simulink model "TBS_SIM"  (R2021a)
settings: Solver=ode5  StartTime=15  StopTime=100  FixedStep=0.002  RelTol=1e-3
PreLoadFcn:
  | TBS_Cai_simu_init_20170316
StopFcn:
  | TBS_SIMULATION_LOG
undefined symbols (not defined in the file): air_density, g, L1X, L2X, L2Y, L3X, L3Y, MAC1, MAC2, MAC3, magnitude, mass, motor_m0, motor_t0, ORIGIN_CD, ORIGIN_CL, ORIGIN_CM, S_seg1, S_seg2, S_seg3
libraries: aerolibconvert2 x20, pid_lib x10, sharedtransform x4, aerolibwind2 x3, simulink x2, shared6dof x1, aerolibasang x1
(part 3 of 3)

== system TBS_SIM/Variant Control System/Transition/Trans/Cruise Controller/Cruise ==
  Ve : Inport
  Xe : Inport  Port=2
  DCM : Inport  Port=3
  pqr : Inport  Port=4
  V_b : Inport  Port=5
  Euler : Inport  Port=6
  Angle Conversion : aerolibconvert2/Angle Conversion  IU=rad  OU=deg
  Demux : Demux
  Demux2 : Demux  Outputs=3
  Mux1 : Mux  Inputs=2
  Mux3 : Mux  Inputs=2
  Saturation : Saturate  UpperLimit=10000  LowerLimit=0
  Saturation1 : Saturate  UpperLimit=10000  LowerLimit=0
  Saturation2 : Saturate  UpperLimit=16.5  LowerLimit=-23
  Saturation3 : Saturate  UpperLimit=16.5  LowerLimit=-23
  Terminator : Terminator
  map : MATLAB Function  TreatAsAtomicUnit=on
  nav : MATLAB Function  TreatAsAtomicUnit=on
  ve : Scope  NumInputPorts=3
  RS : Outport
  "Actuator " : Outport  Port=2
  wires:
  V_b/1 -> nav/3(v)
  map/1(output) -> Demux/1
  Saturation/1 -> Mux1/1
  Demux/1 -> Saturation/1
  Demux/2 -> Saturation1/1
  Saturation1/1 -> Mux1/2
  Saturation2/1 -> Mux3/1
  Demux/4 -> Saturation3/1
  Saturation3/1 -> Mux3/2
  Demux/3 -> Saturation2/1
  nav/1(output) -> map/1(F_des)
  Angle Conversion/1 -> nav/2(PRY)
  Demux2/1 -> ve/1
  Demux2/2 -> ve/2
  Demux2/3 -> ve/3
  Ve/1 -> Demux2/1
  Xe/1 -> nav/1(p)
  pqr/1 -> nav/4(pqr)
  Mux1/1 -> RS/1
  Mux3/1 -> "Actuator "/1
  Euler/1 -> Angle Conversion/1
  DCM/1 -> Terminator/1

== system TBS_SIM/Variant Control System/Transition/Trans/Transition Controller/Hover ==
  Ve : Inport
  Xe : Inport  Port=2
  DCM : Inport  Port=3
  pqr : Inport  Port=4
  des_v : Inport  Port=5
  des_p : Inport  Port=6
  Attitude controller : Subsystem
  Constant1 : Constant  Value=[0,0,0]
  Demux4 : Demux
  Direction Cosine Matrix to Rotation Angles : sharedtransform/Direction Cosine Matrix to Rotation Angles  rotationOrder=YZX  aMode=aMode  action=None  tolerance=eps(2)
      settings: SourceProductBaseCode=AE,PW,DR,MT,UV,VE
  Mux2 : Mux  Inputs=2
  Mux4 : Mux  Inputs=2
  Nav_controller(quad_axes) : Subsystem
  Ramp1 : simulink/Sources/Ramp  slope=18  start=0  InitialOutput=0
  Saturation1 : Saturate  UpperLimit=80
  Saturation4 : Saturate  UpperLimit=10000  LowerLimit=0
  Saturation5 : Saturate  UpperLimit=10000  LowerLimit=0
  Saturation6 : Saturate  UpperLimit=16.5  LowerLimit=-23
  Saturation7 : Saturate  UpperLimit=16.5  LowerLimit=-23
  Scope : Scope  NumInputPorts=2
  Sum : Sum  Inputs=-+|
  map1 : Subsystem
  RS : Outport
  "Actuator " : Outport  Port=2
  wires:
  Saturation6/1 -> Mux4/1
  map1/1(Act) -> Demux4/1
  Mux4/1 -> "Actuator "/1
  Saturation4/1 -> Mux2/1
  Ve/1 -> Nav_controller(quad_axes)/1(True velocity)
  Demux4/2 -> Saturation5/1
  Demux4/4 -> Saturation7/1
  Saturation7/1 -> Mux4/2
  Xe/1 -> Nav_controller(quad_axes)/2(True Position)
  Demux4/1 -> Saturation4/1
  Saturation5/1 -> Mux2/2
  DCM/1 -> Direction Cosine Matrix to Rotation Angles/1
  Nav_controller(quad_axes)/1(phi_des) -> Attitude controller/1(phi_des)
  Attitude controller/2("M_C ") -> map1/2(M_c)
  Demux4/3 -> Saturation6/1
  pqr/1 -> Attitude controller/5(pqr)
  Direction Cosine Matrix to Rotation Angles/1 -> Nav_controller(quad_axes)/5(True PRY), Attitude controller/4(PRY)
  Attitude controller/1(F_c) -> map1/1(F_c)
  Constant1/1 -> Attitude controller/6(des_pqr)
  Nav_controller(quad_axes)/3(F_des) -> Attitude controller/3(F_des)
  Mux2/1 -> RS/1
  des_v/1 -> Nav_controller(quad_axes)/3(Desired velocity)
  des_p/1 -> Nav_controller(quad_axes)/4(Desired Position)
  Saturation1/1 -> Sum/1
  Ramp1/1 -> Saturation1/1
  Nav_controller(quad_axes)/2("theta_des ") -> Scope/2, Sum/2  "before slope"
  Sum/1 -> Scope/1, Attitude controller/2(theta_des)  "Theta_des"

== system TBS_SIM/Variant Control System/Transition/Trans/Transition Controller/Hover/Attitude controller ==
  phi_des : Inport
  theta_des : Inport  Port=2
  F_des : Inport  Port=3
  PRY : Inport  Port=4
  pqr : Inport  Port=5
  des_pqr : Inport  Port=6
  Add : Sum  Inputs=+-
  Angle Conversion1 : aerolibconvert2/Angle Conversion  IU=rad  OU=deg
  Constant1 : Constant  Value=90
  Demux : Demux  Outputs=3
  Gain : Gain  Gain=[-0.05;0.07;0.08]
  Gain1 : Gain  Gain=[-0.4;-0.8;1.4]
  Gain2 : Gain  Gain=[0 0 1; 0 1 0; 1 0 0]  Multiplication=Matrix(K*u)
  Gain3 : Gain  Gain=-1
  Gain4 : Gain  Gain=-1
  Mux : Mux  Inputs=3
  Scope1 : Scope
  Scope2 : Scope
  error_phi : Sum  Inputs=-+
  error_phi1 : Sum  Inputs=-+
  error_pqr : Sum  Inputs=-+
  error_pqr1 : Sum  Inputs=-+
  F_c : Outport
  "M_C " : Outport  Port=2
  wires:
  F_des/1 -> F_c/1
  des_pqr/1 -> error_pqr/1
  pqr/1 -> error_pqr/2
  phi_des/1 -> error_phi/1
  theta_des/1 -> error_phi1/1
  error_phi1/1 -> Mux/2
  Gain/1 -> Add/1
  Gain1/1 -> Scope2/1, Add/2
  PRY/1 -> Angle Conversion1/1
  error_phi/1 -> Mux/1
  Gain4/1 -> Mux/3
  Mux/1 -> Scope1/1, Gain/1
  error_pqr/1 -> Gain2/1
  Gain2/1 -> Gain1/1
  Add/1 -> "M_C "/1
  Demux/2 -> Gain3/1
  Gain3/1 -> error_phi/2
  Demux/1 -> error_pqr1/2
  Constant1/1 -> error_pqr1/1
  error_pqr1/1 -> error_phi1/2
  Angle Conversion1/1 -> Demux/1
  Demux/3 -> Gain4/1

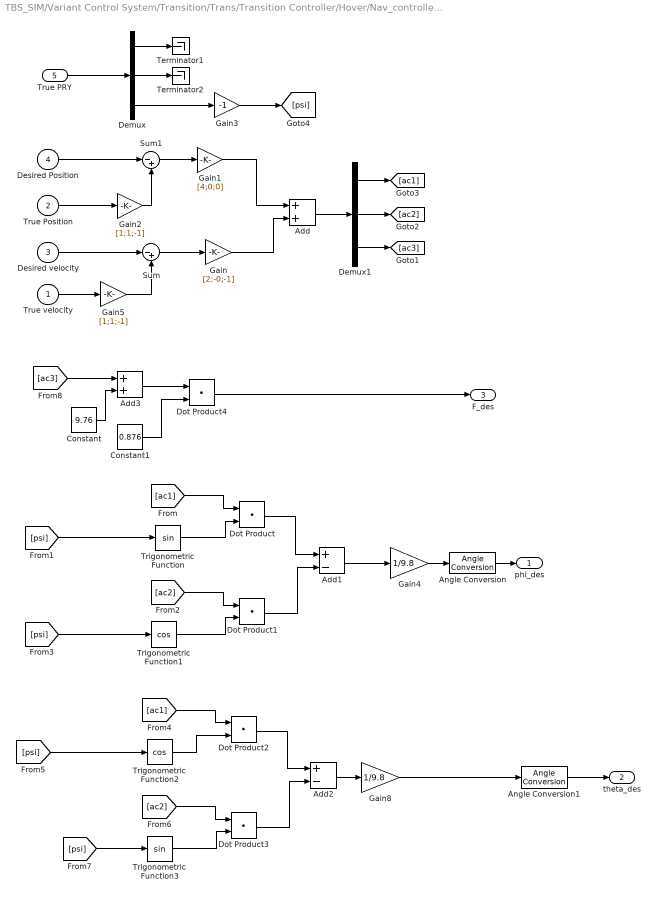
== system TBS_SIM/Variant Control System/Transition/Trans/Transition Controller/Hover/Nav_controller(quad_axes) ==
  True velocity : Inport
  True Position : Inport  Port=2
  Desired velocity : Inport  Port=3
  Desired Position : Inport  Port=4
  True PRY : Inport  Port=5
  Add : Sum
  Add1 : Sum  Inputs=+-
  Add2 : Sum  Inputs=+-
  Add3 : Sum
  Angle Conversion : aerolibconvert2/Angle Conversion  IU=rad  OU=deg
  Angle Conversion1 : aerolibconvert2/Angle Conversion  IU=rad  OU=deg
  Constant : Constant  Value=9.76
  Constant1 : Constant  Value=0.876
  Demux : Demux  Outputs=3
  Demux1 : Demux  Outputs=3
  Dot Product{,1..4} (5 alike) : DotProduct  InputSameDT=on  OutDataTypeStr=Inherit: Inherit via internal rule
  Gain : Gain  Gain=[2;-0;-1]
  Gain1 : Gain  Gain=[4;0;0]
  Gain2 : Gain  Gain=[1;1;-1]
  Gain3 : Gain  Gain=-1
  Gain4 : Gain  Gain=1/9.8
  Gain5 : Gain  Gain=[1;1;-1]
  Gain8 : Gain  Gain=1/9.8
  Sum : Sum  Inputs=|-+
  Sum1 : Sum  Inputs=|-+
  Terminator1 : Terminator
  Terminator2 : Terminator
  Trigonometric Function : Trigonometry
  Trigonometric Function1 : Trigonometry  Operator=cos
  Trigonometric Function2 : Trigonometry  Operator=cos
  Trigonometric Function3 : Trigonometry
  phi_des : Outport
  "theta_des " : Outport  Port=2
  F_des : Outport  Port=3
  wires:
  True velocity/1 -> Gain5/1
  Desired velocity/1 -> Sum/1
  Sum/1 -> Gain/1
  Sum1/1 -> Gain1/1
  Gain1/1 -> Add/1
  Gain/1 -> Add/2
  True PRY/1 -> Demux/1
  Demux/1 -> Terminator1/1
  Demux/3 -> Gain3/1
  Demux/2 -> Terminator2/1
  Add/1 -> Demux1/1
  Demux1/2 -> [ac2]
  [ac1] -> Dot Product/1
  Trigonometric Function/1 -> Dot Product/2
  [psi] -> Trigonometric Function/1
  [ac2] -> Dot Product1/1
  Trigonometric Function1/1 -> Dot Product1/2
  [psi] -> Trigonometric Function1/1
  Dot Product/1 -> Add1/1
  Dot Product1/1 -> Add1/2
  Add1/1 -> Gain4/1
  [ac1] -> Dot Product2/1
  Trigonometric Function2/1 -> Dot Product2/2
  [psi] -> Trigonometric Function2/1
  [ac2] -> Dot Product3/1
  Trigonometric Function3/1 -> Dot Product3/2
  [psi] -> Trigonometric Function3/1
  Dot Product2/1 -> Add2/1
  Dot Product3/1 -> Add2/2
  Add2/1 -> Gain8/1
  [ac3] -> Add3/1
  Constant/1 -> Add3/2
  Add3/1 -> Dot Product4/1
  Constant1/1 -> Dot Product4/2
  Dot Product4/1 -> F_des/1
  Demux1/1 -> [ac1]
  Demux1/3 -> [ac3]
  True Position/1 -> Gain2/1
  Gain2/1 -> Sum1/2
  Desired Position/1 -> Sum1/1
  Gain3/1 -> [psi]
  Gain4/1 -> Angle Conversion/1
  Angle Conversion/1 -> phi_des/1
  Gain8/1 -> Angle Conversion1/1
  Angle Conversion1/1 -> "theta_des "/1
  Gain5/1 -> Sum/2

== system TBS_SIM/Variant Control System/Transition/Trans/Transition Controller/Hover/map1 ==
  F_c : Inport
  M_c : Inport  Port=2
  Constant : Constant  Value=100
  Constant1 : Constant  Value=9.5
  Constant2 : Constant  Value=0.3
  Demux : Demux  Outputs=3
  Gain : Gain  Gain=1000
  Gain1 : Gain  Gain=1000
  Gain2 : Gain  Gain=50
  Gain3 : Gain  Gain=50
  Mux : Mux
  Sum : Sum  Inputs=-+|
  Sum1 : Sum  Inputs=|++
  Sum2 : Sum  Inputs=|+-
  Sum3 : Sum  Inputs=-+|
  Sum4 : Sum  Inputs=|++
  Sum5 : Sum  Inputs=|++
  Sum6 : Sum  Inputs=+-|
  Act : Outport
  wires:
  M_c/1 -> Demux/1
  F_c/1 -> Gain/1
  Demux/1 -> Gain1/1
  Gain1/1 -> Sum/2
  Constant/1 -> Sum/1
  Gain/1 -> Sum2/1, Sum1/1
  Sum/1 -> Sum1/2, Sum2/2
  Sum1/1 -> Mux/1
  Sum2/1 -> Mux/2
  Demux/2 -> Gain2/1
  Demux/3 -> Gain3/1
  Gain3/1 -> Sum4/1
  Constant1/1 -> Sum3/1
  Gain2/1 -> Sum3/2
  Constant2/1 -> Sum4/2
  Mux/1 -> Act/1
  Sum3/1 -> Sum5/1
  Sum4/1 -> Sum6/2, Sum5/2
  Sum5/1 -> Mux/4, Sum6/1
  Sum6/1 -> Mux/3

== stateflow chart TBS_SIM/Variant Control System/Transition/Trans/Chart1 ==
  settings: executeAtInitialization=1
  state Transition
    during:
    trans_mode=1;
  state Cruise
    during:
    trans_mode=0;
  (default) -> Transition
  Transition -> Cruise : [v>2.5&&pitch<=30]
  data: v input; trans_mode output; pitch input

== matlab function TBS_SIM/Variant Control System/Cruise/Cruise/map ==
  data: F_des input; output output
function output  = ac(F_des)
%UNTITLED Summary of this function goes here
%   Detailed explanation goes here
% error_v=des_s(4:6)-s(4:6);
% k_v=[4 0 0;
%     5 0 0;
%     5 0 0];
% F_c=k_v(:,1).*error_v;
rs_mean=F_des(1)*2000;
deltars=F_des(4)*1000-100;
RS1=rs_mean+deltars;
RS2=rs_mean-deltars;
e=F_des(3)*50;
a=F_des(2)*50+0.3;
r=e-a;
l=e+a;
output=[RS1,RS2,r,l];
end

== matlab function TBS_SIM/Variant Control System/Cruise/Cruise/nav ==
  data: p input; PRY input; v input; output output; pqr input
function output   = slx_nav_controller( p,PRY,v,pqr)
%UNTITLED Summary of this function goes here
%   Detailed explanation goes here
height=-p(3);
eh=50-height;
ev=9-v(1);
des_t=4+0*eh+1*ev;
%des_t=2.8;
e_att=[0;8;0]-PRY;
des_M=zeros(3,1);
des_M(1)=0.08*e_att(1)-0.05*pqr(1);
des_M(2)=-0.1*e_att(2)+0.8*pqr(2);
des_M(3)=-0.1*e_att(3)+0.5*pqr(3);
output=[des_t;des_M];
end

== matlab function TBS_SIM/Variant Control System/Transition/Trans/MATLAB Function ==
  data: v input; y output; pitch input
function y = fcn(v,pitch)
    trans_mode=1;
    if v>2.5 && pitch<=30
        trans_mode=0;
    end
y = trans_mode;

== matlab function TBS_SIM/Variant Control System/Transition/Trans/Cruise Controller/Cruise/map ==
  data: F_des input; output output
function output  = ac(F_des)
%UNTITLED Summary of this function goes here
%   Detailed explanation goes here
% error_v=des_s(4:6)-s(4:6);
% k_v=[4 0 0;
%     5 0 0;
%     5 0 0];
% F_c=k_v(:,1).*error_v;
rs_mean=F_des(1)*2000;
deltars=F_des(4)*1000-100;
RS1=rs_mean+deltars;
RS2=rs_mean-deltars;
e=F_des(3)*50;
a=F_des(2)*50+0.3;
r=e-a;
l=e+a;
output=[RS1,RS2,r,l];
end

== matlab function TBS_SIM/Variant Control System/Hover/MATLAB Function ==
  data: out output; t input
function out = fcn(t)
x=0;
y=0;
z=0.01*t;
out=[x y z]';

== matlab function TBS_SIM/Variant Control System/Hover_yaw/MATLAB Function ==
  data: out output; t input
function out = fcn(t)
x=0;
y=0;
z=-0.5*t;
out=[x y z]';

== matlab function TBS_SIM/Variant Control System/Transition/Trans/Cruise Controller/Cruise/nav ==
  data: p input; PRY input; v input; output output; pqr input
function output   = slx_nav_controller( p,PRY,v,pqr)
%UNTITLED Summary of this function goes here
%   Detailed explanation goes here
height=-p(3);
eh=50-height;
ev=9-v(1);
des_t=4+0*eh+1*ev;
%des_t=2.8;
e_att=[0;8;0]-PRY;
des_M=zeros(3,1);
des_M(1)=0.08*e_att(1)-0.05*pqr(1);
des_M(2)=-0.1*e_att(2)+0.8*pqr(2);
des_M(3)=-0.1*e_att(3)+0.5*pqr(3);
output=[des_t;des_M];
end
